simulink model "DcGearmotor"  (R2022b)
settings: Solver=VariableStepAuto  StartTime=0.0  StopTime=20  RelTol=1e-3
values from neighbouring files (symbols this model uses):
  degs2rpm = 0.166666666667    [parameters.mat]
  drv =     [parameters.mat]
  gbox =     [parameters.mat]
  hub =     [parameters.mat]
  joint =     [parameters.mat]
  mld =     [parameters.mat]
  mot =     [parameters.mat]
  rads2rpm = 9.54929658551    [parameters.mat]
  real =     [parameters.mat]
  sens =     [parameters.mat]
  Ts = 0.001    [parameters.mat]
undefined symbols (not defined in the file or in its folder): der, pid, simul
settings Model: Creator=emanuelevitetta  LastModifiedBy=emanuelevitetta

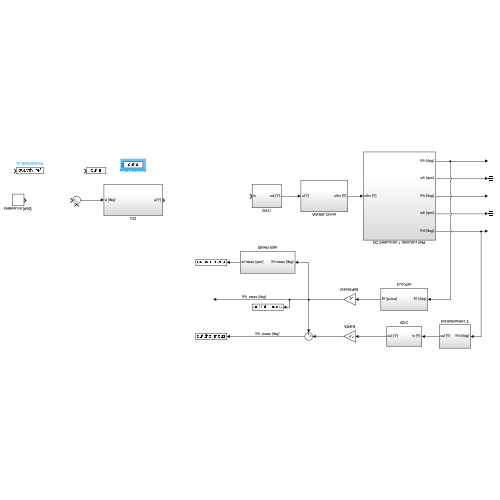
[thumbnail: Simulink's stored preview of the top-level diagram]
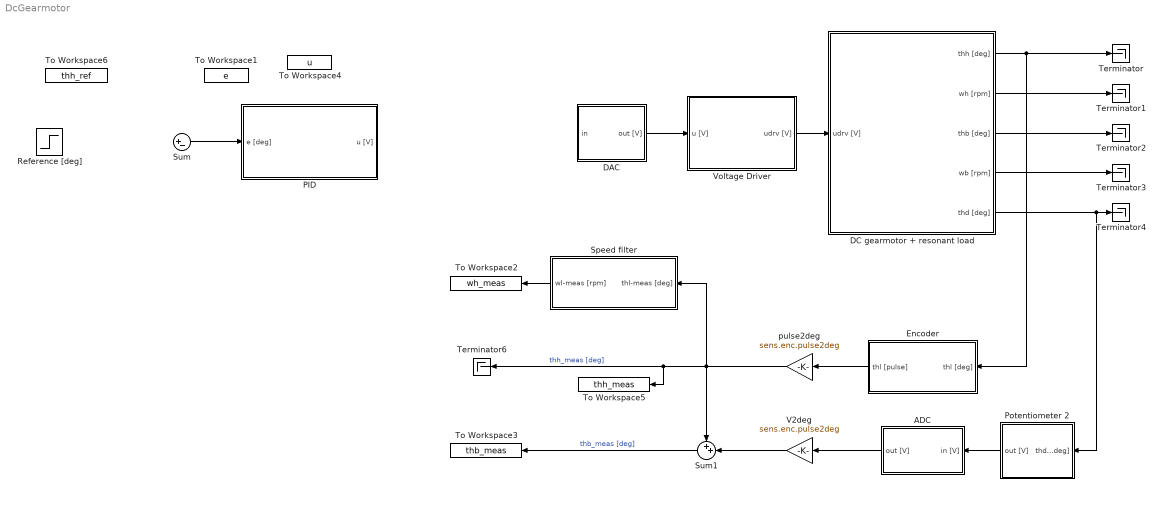
== system DcGearmotor ==
  ADC : Subsystem
  DAC : Subsystem
  DC gearmotor + resonant load : Subsystem
  Encoder : Subsystem
  PID : Subsystem
  Potentiometer 2 : Subsystem
  Reference [deg] : Step  After=simul.stepdeg
  Speed filter : Subsystem
  Sum : Sum  Inputs=|+-
  Sum1 : Sum  Inputs=++|
  Terminator{,1..4,6} (6 alike) : Terminator
  To Workspace1 : ToWorkspace  VariableName=e  SaveFormat=Timeseries  SampleTime=-1
  To Workspace2 : ToWorkspace  VariableName=wh_meas  SaveFormat=Timeseries  SampleTime=Ts
  To Workspace3 : ToWorkspace  VariableName=thb_meas  SaveFormat=Timeseries  SampleTime=Ts
  To Workspace4 : ToWorkspace  VariableName=u  SaveFormat=Timeseries  SampleTime=Ts
  To Workspace5 : ToWorkspace  VariableName=thh_meas  SaveFormat=Timeseries  SampleTime=Ts
  To Workspace6 : ToWorkspace  VariableName=thh_ref  SaveFormat=Timeseries  SampleTime=-1
  V2deg : Gain  Gain=sens.enc.pulse2deg
  Voltage Driver : Subsystem
  pulse2deg : Gain  Gain=sens.enc.pulse2deg
  wires:
  Voltage Driver/1(udrv [V]) -> DC gearmotor + resonant load/1(udrv [V])
  DAC/1(out [V]) -> Voltage Driver/1(u [V])
  Sum/1 -> PID/1(e [deg])
  DC gearmotor + resonant load/1(thh [deg]) -> Encoder/1(thl [deg]), Terminator/1
  DC gearmotor + resonant load/2(wh [rpm]) -> Terminator1/1
  DC gearmotor + resonant load/3(thb [deg]) -> Terminator2/1
  DC gearmotor + resonant load/4(wb [rpm]) -> Terminator3/1
  DC gearmotor + resonant load/5(thd [deg]) -> Potentiometer 2/1(thd [deg]), Terminator4/1
  Potentiometer 2/1(out [V]) -> ADC/1(in [V])
  Encoder/1(thl [pulse]) -> pulse2deg/1
  ADC/1(out [V]) -> V2deg/1
  V2deg/1 -> Sum1/2
  Speed filter/1(wl-meas [rpm]) -> To Workspace2/1
  pulse2deg/1 -> Speed filter/1(thl-meas [deg]), Terminator6/1, To Workspace5/1, Sum1/1  "thh_meas [deg]"
  Sum1/1 -> To Workspace3/1  "thb_meas [deg]"

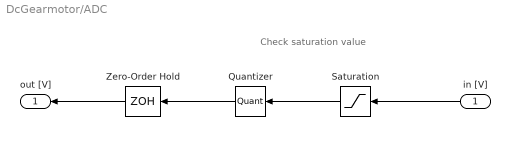
== system DcGearmotor/ADC ==
  note: Check saturation value
  in [V] : Inport
  Quantizer : Quantizer  QuantizationInterval=daq.adc.q
  Saturation : Saturate  UpperLimit=10  LowerLimit=-10
  Zero-Order Hold : ZeroOrderHold  SampleTime=Ts
  out [V] : Outport
  wires:
  in [V]/1 -> Saturation/1
  Saturation/1 -> Quantizer/1
  Zero-Order Hold/1 -> out [V]/1
  Quantizer/1 -> Zero-Order Hold/1

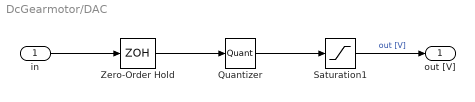
== system DcGearmotor/DAC ==
  in : Inport
  Quantizer : Quantizer  QuantizationInterval=daq.dac.q
  Saturation1 : Saturate  UpperLimit=10  LowerLimit=-10
  Zero-Order Hold : ZeroOrderHold  SampleTime=Ts
  out [V] : Outport
  wires:
  Saturation1/1 -> out [V]/1  "out [V]"
  in/1 -> Zero-Order Hold/1
  Zero-Order Hold/1 -> Quantizer/1
  Quantizer/1 -> Saturation1/1

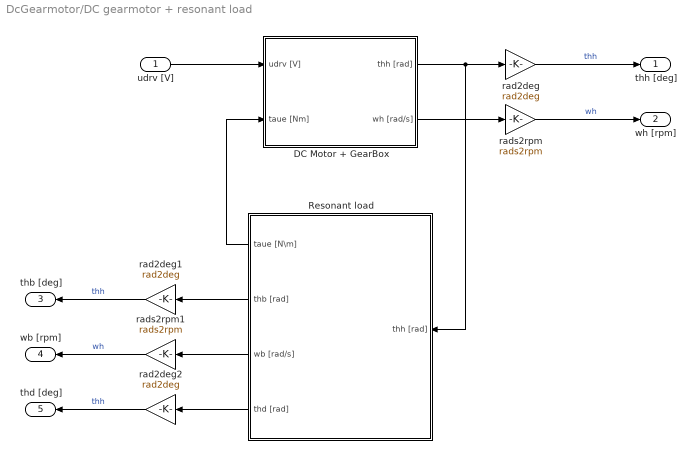
== system DcGearmotor/DC gearmotor + resonant load ==
  udrv [V] : Inport
  DC Motor + GearBox : Subsystem
  Resonant load : Subsystem
  rad2deg : Gain  Gain=rad2deg
  rad2deg1 : Gain  Gain=rad2deg
  rad2deg2 : Gain  Gain=rad2deg
  rads2rpm : Gain  Gain=rads2rpm
  rads2rpm1 : Gain  Gain=rads2rpm
  thh [deg] : Outport
  wh [rpm] : Outport  Port=2
  thb [deg] : Outport  Port=3
  wb [rpm] : Outport  Port=4
  thd [deg] : Outport  Port=5
  wires:
  rads2rpm/1 -> wh [rpm]/1  "wh"
  Resonant load/1(taue [N\m]) -> DC Motor + GearBox/2(taue [Nm])
  Resonant load/4(thd [rad]) -> rad2deg2/1
  rads2rpm1/1 -> wb [rpm]/1  "wh"
  DC Motor + GearBox/1(thh [rad]) -> Resonant load/1(thh [rad]), rad2deg/1
  udrv [V]/1 -> DC Motor + GearBox/1(udrv [V])
  rad2deg1/1 -> thb [deg]/1  "thh"
  Resonant load/3(wb [rad/s]) -> rads2rpm1/1
  DC Motor + GearBox/2(wh [rad/s]) -> rads2rpm/1
  rad2deg/1 -> thh [deg]/1  "thh"
  Resonant load/2(thb [rad]) -> rad2deg1/1
  rad2deg2/1 -> thd [deg]/1  "thh"

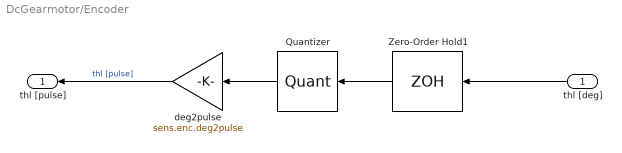
== system DcGearmotor/Encoder ==
  thl [deg] : Inport
  Quantizer : Quantizer  QuantizationInterval=sens.enc.pulse2deg
  Zero-Order Hold1 : ZeroOrderHold  SampleTime=Ts
  deg2pulse : Gain  Gain=sens.enc.deg2pulse
  thl [pulse] : Outport
  wires:
  thl [deg]/1 -> Zero-Order Hold1/1
  Zero-Order Hold1/1 -> Quantizer/1
  deg2pulse/1 -> thl [pulse]/1  "thl [pulse]"
  Quantizer/1 -> deg2pulse/1

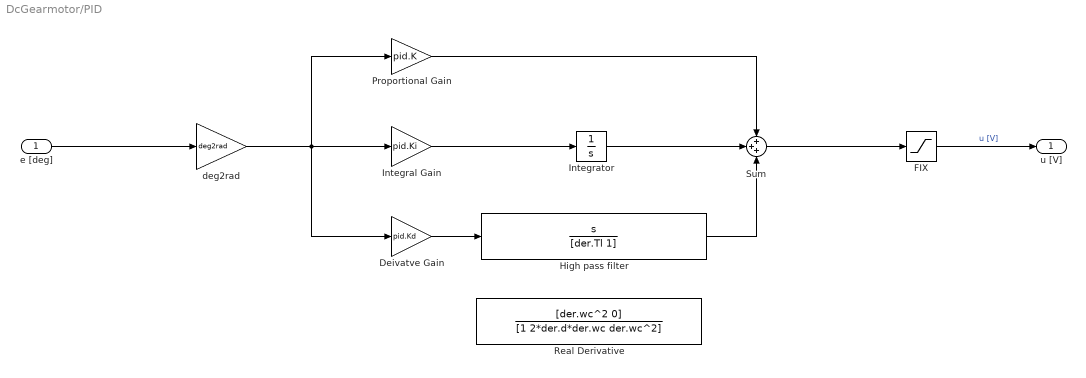
== system DcGearmotor/PID ==
  e [deg] : Inport
  Deivatve Gain : Gain  Gain=pid.Kd
  "FIX " : Saturate  UpperLimit=10  LowerLimit=-10
  High pass filter : TransferFcn  Numerator=[1 0]  Denominator=[der.Tl 1]
  Integral Gain : Gain  Gain=pid.Ki
  Integrator : Integrator
  Proportional Gain : Gain  Gain=pid.K
  Real Derivative : TransferFcn  Numerator=[der.wc^2 0]  Denominator=[1 2*der.d*der.wc der.wc^2]
  Sum : Sum  Inputs=+++
  deg2rad : Gain  Gain=deg2rad
  u [V] : Outport
  wires:
  Deivatve Gain/1 -> High pass filter/1
  e [deg]/1 -> deg2rad/1
  Integrator/1 -> Sum/2
  "FIX "/1 -> u [V]/1  "u [V]"
  deg2rad/1 -> Deivatve Gain/1, Proportional Gain/1, Integral Gain/1
  High pass filter/1 -> Sum/3
  Integral Gain/1 -> Integrator/1
  Proportional Gain/1 -> Sum/1
  Sum/1 -> "FIX "/1

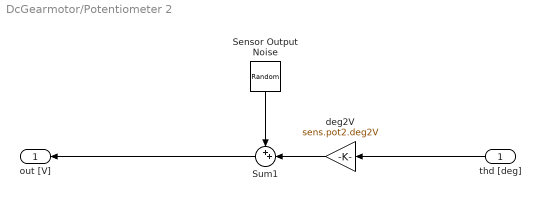
== system DcGearmotor/Potentiometer 2 ==
  thd [deg] : Inport
  Sensor Output Noise : RandomNumber  Variance=sens.pot2.var  SampleTime=0.1
  Sum1 : Sum  Inputs=++|
  deg2V : Gain  Gain=sens.pot2.deg2V
  out [V] : Outport
  wires:
  Sum1/1 -> out [V]/1
  thd [deg]/1 -> deg2V/1
  Sensor Output Noise/1 -> Sum1/1
  deg2V/1 -> Sum1/2

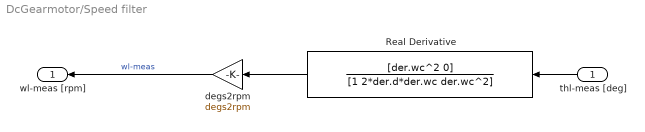
== system DcGearmotor/Speed filter ==
  thl-meas [deg] : Inport
  Real Derivative : TransferFcn  Numerator=[der.wc^2 0]  Denominator=[1 2*der.d*der.wc der.wc^2]
  degs2rpm : Gain  Gain=degs2rpm
  wl-meas [rpm] : Outport
  wires:
  thl-meas [deg]/1 -> Real Derivative/1
  degs2rpm/1 -> wl-meas [rpm]/1  "wl-meas"
  Real Derivative/1 -> degs2rpm/1

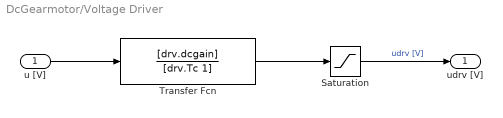
== system DcGearmotor/Voltage Driver ==
  u [V] : Inport
  Saturation : Saturate  UpperLimit=12  LowerLimit=-12
  Transfer Fcn : TransferFcn  Numerator=[drv.dcgain]  Denominator=[drv.Tc 1]
  udrv [V] : Outport
  wires:
  Saturation/1 -> udrv [V]/1  "udrv [V]"
  u [V]/1 -> Transfer Fcn/1
  Transfer Fcn/1 -> Saturation/1

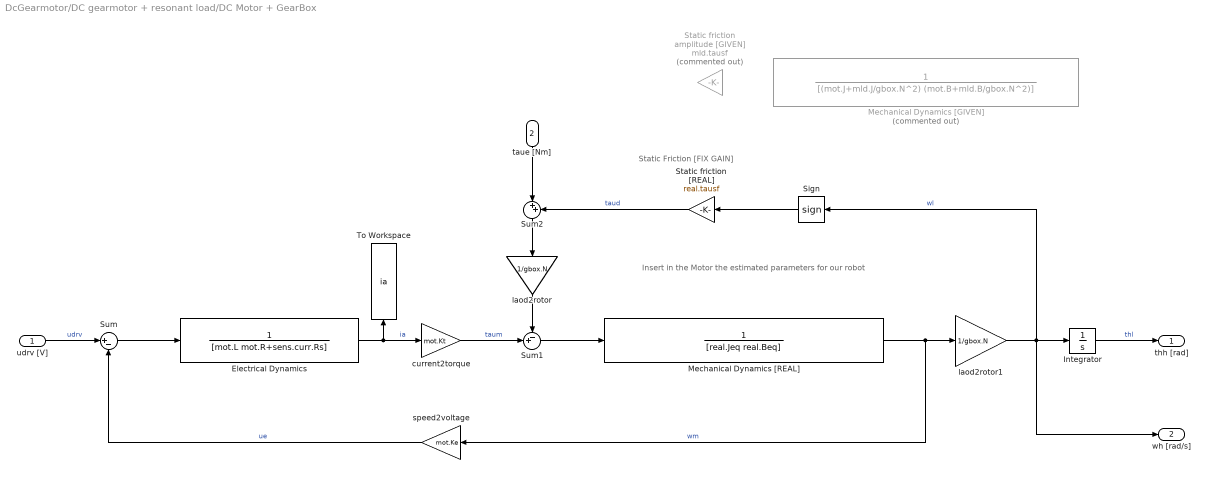
== system DcGearmotor/DC gearmotor + resonant load/DC Motor + GearBox ==
  note: Insert in the Motor the estimated parameters for our robot
  note: Static Friction [FIX GAIN]
  udrv [V] : Inport
  taue [Nm] : Inport  Port=2
  Electrical Dynamics : TransferFcn  Denominator=[mot.L mot.R+sens.curr.Rs]
  Integrator : Integrator
  Mechanical Dynamics [GIVEN] : TransferFcn  Commented=on  Denominator=[(mot.J+mld.J/gbox.N^2) (mot.B+mld.B/gbox.N^2)]
  Mechanical Dynamics [REAL] : TransferFcn  Denominator=[real.Jeq real.Beq]
  Sign : Signum  ZeroCross=off
  Static friction [REAL] : Gain  Gain=real.tausf
  Static friction amplitude [GIVEN] : Gain  Commented=on  Gain=mld.tausf
  Sum : Sum  Inputs=|+-
  Sum1 : Sum  Inputs=-+|
  Sum2 : Sum  Inputs=|++
  To Workspace : ToWorkspace  VariableName=ia  SaveFormat=Timeseries  SampleTime=-1
  current2torque : Gain  Gain=mot.Kt
  laod2rotor : Gain  Gain=1/gbox.N
  laod2rotor1 : Gain  Gain=1/gbox.N
  speed2voltage : Gain  Gain=mot.Ke
  thh [rad] : Outport
  wh [rad/s] : Outport  Port=2
  wires:
  Sign/1 -> Static friction [REAL]/1
  Electrical Dynamics/1 -> To Workspace/1, current2torque/1  "ia"
  Sum1/1 -> Mechanical Dynamics [REAL]/1
  laod2rotor1/1 -> wh [rad/s]/1, Sign/1, Integrator/1  "wl"
  laod2rotor/1 -> Sum1/1
  udrv [V]/1 -> Sum/1  "udrv"
  current2torque/1 -> Sum1/2  "taum"
  speed2voltage/1 -> Sum/2  "ue"
  Sum/1 -> Electrical Dynamics/1
  Mechanical Dynamics [REAL]/1 -> speed2voltage/1, laod2rotor1/1  "wm"
  Sum2/1 -> laod2rotor/1
  Static friction [REAL]/1 -> Sum2/2  "taud"
  taue [Nm]/1 -> Sum2/1
  Integrator/1 -> thh [rad]/1  "thl"

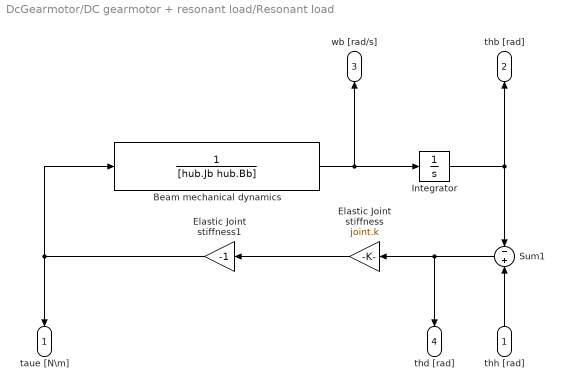
== system DcGearmotor/DC gearmotor + resonant load/Resonant load ==
  thh [rad] : Inport
  Beam mechanical dynamics : TransferFcn  Denominator=[hub.Jb hub.Bb]
  Elastic Joint stiffness : Gain  Gain=joint.k
  Elastic Joint stiffness1 : Gain  Gain=-1
  Integrator : Integrator
  Sum1 : Sum  Inputs=-+
  taue [N\m] : Outport
  thb [rad] : Outport  Port=2
  wb [rad/s] : Outport  Port=3
  thd [rad] : Outport  Port=4
  wires:
  thh [rad]/1 -> Sum1/2
  Beam mechanical dynamics/1 -> wb [rad/s]/1, Integrator/1
  Sum1/1 -> thd [rad]/1, Elastic Joint stiffness/1
  Elastic Joint stiffness/1 -> Elastic Joint stiffness1/1
  Elastic Joint stiffness1/1 -> Beam mechanical dynamics/1, taue [N\m]/1
  Integrator/1 -> thb [rad]/1, Sum1/1
